simulink model "JointSpaceControl_BestInertia"  (R2013a)
settings: Solver=ode3  StartTime=0.0  StopTime=sim_end  FixedStep=0.004  MaxStep=0.008  RelTol=1e-3
PreLoadFcn:
  | Initialization
InitFcn:
  | Initialization
values from neighbouring files (symbols this model uses):
  a_max = [27 27 27 27 27 27]    [Initialization.m]
  dq_0 = qd_actual.signals.values(1,:)    [Initialization.m]
  K_0 = [K0_11, zeros(3,3); zeros(3,3),omega_P_small^2*eye(3,3)]    [Initialization.m]    (also in Plot_PD_Estimation.m)
  K_1 = [K1_11, zeros(3,3); zeros(3,3),2*omega_D_small*eye(3,3)]    [Initialization.m]    (also in Plot_PD_Estimation.m)
  q_0 = q_actual.signals.values(1,:)    [Initialization.m]
  q_max = 2*pi*ones(1,6)    [Initialization.m]
  q_min = -2*pi*ones(1,6)    [Initialization.m]
  torque_max = [150 150 150 28 28 28]    [Initialization.m]
  v_max = 3.4*ones(1,6)    [Initialization.m]
libraries: dsparch4 x30, simulink x2
(part 2 of 3)

== matlab function JointSpaceControl_BestInertia/base_tool_transformation_matrix1 ==
  data: d output; q input; R output
function [d, R]   = base_tool_transformation(q)
% BASE_TOOL_TRANSFORMATION - Transformationmatrix from Base to Tool.
%  Calculates the Base-Tool Transformation matrix based on the current
%  joint positions and returns the rotation matrix and the displacement
%  vector.

theta1 = q(1);
theta2 = q(2);
theta3 = q(3);
theta4 = q(4);
theta5 = q(5);
theta6 = q(6);

theta_1 = theta1;
theta_2 = theta2;
theta_3 = theta3;
theta_4 = theta4;
theta_5 = theta5;
theta_6 = theta6;

% With transformation to accelerometer
T = [[   cos(theta_6)*(sin(theta_1)*sin(theta_5) - cos(theta_5)*(cos(theta_4)*(cos(theta_1)*sin(theta_2)*sin(theta_3) - cos(theta_1)*cos(theta_2)*cos(theta_3)) + sin(theta_4)*(cos(theta_1)*cos(theta_2)*sin(theta_3) + cos(theta_1)*cos(theta_3)*sin(theta_2)))) - sin(theta_6)*(cos(theta_4)*(cos(theta_1)*cos(theta_2)*sin(theta_3) + cos(theta_1)*cos(theta_3)*sin(theta_2)) - sin(theta_4)*(cos(theta_1)*sin(theta_2)*sin(theta_3) - cos(theta_1)*cos(theta_2)*cos(theta_3))), - sin(theta_6)*(sin(theta_1)*sin(theta_5) - cos(theta_5)*(cos(theta_4)*(cos(theta_1)*sin(theta_2)*sin(theta_3) - cos(theta_1)*cos(theta_2)*cos(theta_3)) + sin(theta_4)*(cos(theta_1)*cos(theta_2)*sin(theta_3) + cos(theta_1)*cos(theta_3)*sin(theta_2)))) - cos(theta_6)*(cos(theta_4)*(cos(theta_1)*cos(theta_2)*sin(theta_3) + cos(theta_1)*cos(theta_3)*sin(theta_2)) - sin(theta_4)*(cos(theta_1)*sin(theta_2)*sin(theta_3) - cos(theta_1)*cos(theta_2)*cos(theta_3))), cos(theta_5)*sin(theta_1) + sin(theta_5)*(cos(theta_4)*(cos(theta_1)*sin(theta_2)*sin(theta_3) - cos(theta_1)*cos(theta_2)*cos(theta_3)) + sin(theta_4)*(cos(theta_1)*cos(theta_2)*sin(theta_3) + cos(theta_1)*cos(theta_3)*sin(theta_2))), (109*sin(theta_1))/1000 - (17*cos(theta_1)*cos(theta_2))/40 + (183*cos(theta_5)*sin(theta_1))/2000 + (347*cos(theta_6)*(sin(theta_1)*sin(theta_5) - cos(theta_5)*(cos(theta_4)*(cos(theta_1)*sin(theta_2)*sin(theta_3) - cos(theta_1)*cos(theta_2)*cos(theta_3)) + sin(theta_4)*(cos(theta_1)*cos(theta_2)*sin(theta_3) + cos(theta_1)*cos(theta_3)*sin(theta_2)))))/20000 + (93*cos(theta_4)*(cos(theta_1)*cos(theta_2)*sin(theta_3) + cos(theta_1)*cos(theta_3)*sin(theta_2)))/1000 - (121*sin(theta_6)*(sin(theta_1)*sin(theta_5) - cos(theta_5)*(cos(theta_4)*(cos(theta_1)*sin(theta_2)*sin(theta_3) - cos(theta_1)*cos(theta_2)*cos(theta_3)) + sin(theta_4)*(cos(theta_1)*cos(theta_2)*sin(theta_3) + cos(theta_1)*cos(theta_3)*sin(theta_2)))))/20000 - (93*sin(theta_4)*(cos(theta_1)*sin(theta_2)*sin(theta_3) - cos(theta_1)*cos(theta_2)*cos(theta_3)))/1000 - (121*cos(theta_6)*(cos(theta_4)*(cos(theta_1)*cos(theta_2)*sin(theta_3) + cos(theta_1)*cos(theta_3)*sin(theta_2)) - sin(theta_4)*(cos(theta_1)*sin(theta_2)*sin(theta_3) - cos(theta_1)*cos(theta_2)*cos(theta_3))))/20000 + (183*sin(theta_5)*(cos(theta_4)*(cos(theta_1)*sin(theta_2)*sin(theta_3) - cos(theta_1)*cos(theta_2)*cos(theta_3)) + sin(theta_4)*(cos(theta_1)*cos(theta_2)*sin(theta_3) + cos(theta_1)*cos(theta_3)*sin(theta_2))))/2000 - (347*sin(theta_6)*(cos(theta_4)*(cos(theta_1)*cos(theta_2)*sin(theta_3) + cos(theta_1)*cos(theta_3)*sin(theta_2)) - sin(theta_4)*(cos(theta_1)*sin(theta_2)*sin(theta_3) - cos(theta_1)*cos(theta_2)*cos(theta_3))))/20000 + (39243*cos(theta_1)*sin(theta_2)*sin(theta_3))/100000 - (39243*cos(theta_1)*cos(theta_2)*cos(theta_3))/100000]; 
    [ - cos(theta_6)*(cos(theta_1)*sin(theta_5) + cos(theta_5)*(cos(theta_4)*(sin(theta_1)*sin(theta_2)*sin(theta_3) - cos(theta_2)*cos(theta_3)*sin(theta_1)) + sin(theta_4)*(cos(theta_2)*sin(theta_1)*sin(theta_3) + cos(theta_3)*sin(theta_1)*sin(theta_2)))) - sin(theta_6)*(cos(theta_4)*(cos(theta_2)*sin(theta_1)*sin(theta_3) + cos(theta_3)*sin(theta_1)*sin(theta_2)) - sin(theta_4)*(sin(theta_1)*sin(theta_2)*sin(theta_3) - cos(theta_2)*cos(theta_3)*sin(theta_1))),   sin(theta_6)*(cos(theta_1)*sin(theta_5) + cos(theta_5)*(cos(theta_4)*(sin(theta_1)*sin(theta_2)*sin(theta_3) - cos(theta_2)*cos(theta_3)*sin(theta_1)) + sin(theta_4)*(cos(theta_2)*sin(theta_1)*sin(theta_3) + cos(theta_3)*sin(theta_1)*sin(theta_2)))) - cos(theta_6)*(cos(theta_4)*(cos(theta_2)*sin(theta_1)*sin(theta_3) + cos(theta_3)*sin(theta_1)*sin(theta_2)) - sin(theta_4)*(sin(theta_1)*sin(theta_2)*sin(theta_3) - cos(theta_2)*cos(theta_3)*sin(theta_1))), sin(theta_5)*(cos(theta_4)*(sin(theta_1)*sin(theta_2)*sin(theta_3) - cos(theta_2)*cos(theta_3)*sin(theta_1)) + sin(theta_4)*(cos(theta_2)*sin(theta_1)*sin(theta_3) + cos(theta_3)*sin(theta_1)*sin(theta_2))) - cos(theta_1)*cos(theta_5), (93*cos(theta_4)*(cos(theta_2)*sin(theta_1)*sin(theta_3) + cos(theta_3)*sin(theta_1)*sin(theta_2)))/1000 - (183*cos(theta_1)*cos(theta_5))/2000 - (17*cos(theta_2)*sin(theta_1))/40 - (109*cos(theta_1))/1000 - (347*cos(theta_6)*(cos(theta_1)*sin(theta_5) + cos(theta_5)*(cos(theta_4)*(sin(theta_1)*sin(theta_2)*sin(theta_3) - cos(theta_2)*cos(theta_3)*sin(theta_1)) + sin(theta_4)*(cos(theta_2)*sin(theta_1)*sin(theta_3) + cos(theta_3)*sin(theta_1)*sin(theta_2)))))/20000 - (93*sin(theta_4)*(sin(theta_1)*sin(theta_2)*sin(theta_3) - cos(theta_2)*cos(theta_3)*sin(theta_1)))/1000 + (121*sin(theta_6)*(cos(theta_1)*sin(theta_5) + cos(theta_5)*(cos(theta_4)*(sin(theta_1)*sin(theta_2)*sin(theta_3) - cos(theta_2)*cos(theta_3)*sin(theta_1)) + sin(theta_4)*(cos(theta_2)*sin(theta_1)*sin(theta_3) + cos(theta_3)*sin(theta_1)*sin(theta_2)))))/20000 - (121*cos(theta_6)*(cos(theta_4)*(cos(theta_2)*sin(theta_1)*sin(theta_3) + cos(theta_3)*sin(theta_1)*sin(theta_2)) - sin(theta_4)*(sin(theta_1)*sin(theta_2)*sin(theta_3) - cos(theta_2)*cos(theta_3)*sin(theta_1))))/20000 + (183*sin(theta_5)*(cos(theta_4)*(sin(theta_1)*sin(theta_2)*sin(theta_3) - cos(theta_2)*cos(theta_3)*sin(theta_1)) + sin(theta_4)*(cos(theta_2)*sin(theta_1)*sin(theta_3) + cos(theta_3)*sin(theta_1)*sin(theta_2))))/2000 - (347*sin(theta_6)*(cos(theta_4)*(cos(theta_2)*sin(theta_1)*sin(theta_3) + cos(theta_3)*sin(theta_1)*sin(theta_2)) - sin(theta_4)*(sin(theta_1)*sin(theta_2)*sin(theta_3) - cos(theta_2)*cos(theta_3)*sin(theta_1))))/20000 + (39243*sin(theta_1)*sin(theta_2)*sin(theta_3))/100000 - (39243*cos(theta_2)*cos(theta_3)*sin(theta_1))/100000]; 
    [                                                                                                                                         sin(theta_6)*(cos(theta_4)*(cos(theta_2)*cos(theta_3) - sin(theta_2)*sin(theta_3)) - sin(theta_4)*(cos(theta_2)*sin(theta_3) + cos(theta_3)*sin(theta_2))) + cos(theta_5)*cos(theta_6)*(cos(theta_4)*(cos(theta_2)*sin(theta_3) + cos(theta_3)*sin(theta_2)) + sin(theta_4)*(cos(theta_2)*cos(theta_3) - sin(theta_2)*sin(theta_3))),                                                                                                                                         cos(theta_6)*(cos(theta_4)*(cos(theta_2)*cos(theta_3) - sin(theta_2)*sin(theta_3)) - sin(theta_4)*(cos(theta_2)*sin(theta_3) + cos(theta_3)*sin(theta_2))) - cos(theta_5)*sin(theta_6)*(cos(theta_4)*(cos(theta_2)*sin(theta_3) + cos(theta_3)*sin(theta_2)) + sin(theta_4)*(cos(theta_2)*cos(theta_3) - sin(theta_2)*sin(theta_3))),                                                                                -sin(theta_5)*(cos(theta_4)*(cos(theta_2)*sin(theta_3) + cos(theta_3)*sin(theta_2)) + sin(theta_4)*(cos(theta_2)*cos(theta_3) - sin(theta_2)*sin(theta_3))),                                                                                                                                                                                                                                                                                                                                                                                                                                                                                  (121*cos(theta_6)*(cos(theta_4)*(cos(theta_2)*cos(theta_3) - sin(theta_2)*sin(theta_3)) - sin(theta_4)*(cos(theta_2)*sin(theta_3) + cos(theta_3)*sin(theta_2))))/20000 - (39243*cos(theta_2)*sin(theta_3))/100000 - (39243*cos(theta_3)*sin(theta_2))/100000 - (17*sin(theta_2))/40 - (183*sin(theta_5)*(cos(theta_4)*(cos(theta_2)*sin(theta_3) + cos(theta_3)*sin(theta_2)) + sin(theta_4)*(cos(theta_2)*cos(theta_3) - sin(theta_2)*sin(theta_3))))/2000 + (347*sin(theta_6)*(cos(theta_4)*(cos(theta_2)*cos(theta_3) - sin(theta_2)*sin(theta_3)) - sin(theta_4)*(cos(theta_2)*sin(theta_3) + cos(theta_3)*sin(theta_2))))/20000 - (93*cos(theta_4)*(cos(theta_2)*cos(theta_3) - sin(theta_2)*sin(theta_3)))/1000 + (93*sin(theta_4)*(cos(theta_2)*sin(theta_3) + cos(theta_3)*sin(theta_2)))/1000 + (347*cos(theta_5)*cos(theta_6)*(cos(theta_4)*(cos(theta_2)*sin(theta_3) + cos(theta_3)*sin(theta_2)) + sin(theta_4)*(cos(theta_2)*cos(theta_3) - sin(theta_2)*sin(theta_3))))/20000 - (121*cos(theta_5)*sin(theta_6)*(cos(theta_4)*(cos(theta_2)*sin(theta_3) + cos(theta_3)*sin(theta_2)) + sin(theta_4)*(cos(theta_2)*cos(theta_3) - sin(theta_2)*sin(theta_3))))/20000 + 223/2500]; 
    [                                                                                                                                                                                                                                                                                                                                                                                                                                                                            0,                                                                                                                                                                                                                                                                                                                                                                                                                                                                            0,                                                                                                                                                                                                                                          0,                                                                                                                                                                                                                                                                                                                                                                                                                                                                                                                                                                                                                                                                                                                                                                                                                                                                                                                                                                                                                                                                                                                                                                                                                                                                                                                                                                                                                                                                                                                                                                                                                                                                              1]];


% T =  [[cos(theta_6)*(sin(theta_1)*sin(theta_5) - cos(theta_5)*(cos(theta_4)*(cos(theta_1)*sin(theta_2)*sin(theta_3) - cos(theta_1)*cos(theta_2)*cos(theta_3)) + sin(theta_4)*(cos(theta_1)*cos(theta_2)*sin(theta_3) + cos(theta_1)*cos(theta_3)*sin(theta_2)))) - sin(theta_6)*(cos(theta_4)*(cos(theta_1)*cos(theta_2)*sin(theta_3) + cos(theta_1)*cos(theta_3)*sin(theta_2)) - sin(theta_4)*(cos(theta_1)*sin(theta_2)*sin(theta_3) - cos(theta_1)*cos(theta_2)*cos(theta_3))), - sin(theta_6)*(sin(theta_1)*sin(theta_5) - cos(theta_5)*(cos(theta_4)*(cos(theta_1)*sin(theta_2)*sin(theta_3) - cos(theta_1)*cos(theta_2)*cos(theta_3)) + sin(theta_4)*(cos(theta_1)*cos(theta_2)*sin(theta_3) + cos(theta_1)*cos(theta_3)*sin(theta_2)))) - cos(theta_6)*(cos(theta_4)*(cos(theta_1)*cos(theta_2)*sin(theta_3) + cos(theta_1)*cos(theta_3)*sin(theta_2)) - sin(theta_4)*(cos(theta_1)*sin(theta_2)*sin(theta_3) - cos(theta_1)*cos(theta_2)*cos(theta_3))), cos(theta_5)*sin(theta_1) + sin(theta_5)*(cos(theta_4)*(cos(theta_1)*sin(theta_2)*sin(theta_3) - cos(theta_1)*cos(theta_2)*cos(theta_3)) + sin(theta_4)*(cos(theta_1)*cos(theta_2)*sin(theta_3) + cos(theta_1)*cos(theta_3)*sin(theta_2))), (109*sin(theta_1))/1000 - (17*cos(theta_1)*cos(theta_2))/40 + (41*cos(theta_5)*sin(theta_1))/500 + (93*cos(theta_4)*(cos(theta_1)*cos(theta_2)*sin(theta_3) + cos(theta_1)*cos(theta_3)*sin(theta_2)))/1000 - (93*sin(theta_4)*(cos(theta_1)*sin(theta_2)*sin(theta_3) - cos(theta_1)*cos(theta_2)*cos(theta_3)))/1000 + (41*sin(theta_5)*(cos(theta_4)*(cos(theta_1)*sin(theta_2)*sin(theta_3) - cos(theta_1)*cos(theta_2)*cos(theta_3)) + sin(theta_4)*(cos(theta_1)*cos(theta_2)*sin(theta_3) + cos(theta_1)*cos(theta_3)*sin(theta_2))))/500 + (39243*cos(theta_1)*sin(theta_2)*sin(theta_3))/100000 - (39243*cos(theta_1)*cos(theta_2)*cos(theta_3))/100000];
%      [ - cos(theta_6)*(cos(theta_1)*sin(theta_5) + cos(theta_5)*(cos(theta_4)*(sin(theta_1)*sin(theta_2)*sin(theta_3) - cos(theta_2)*cos(theta_3)*sin(theta_1)) + sin(theta_4)*(cos(theta_2)*sin(theta_1)*sin(theta_3) + cos(theta_3)*sin(theta_1)*sin(theta_2)))) - sin(theta_6)*(cos(theta_4)*(cos(theta_2)*sin(theta_1)*sin(theta_3) + cos(theta_3)*sin(theta_1)*sin(theta_2)) - sin(theta_4)*(sin(theta_1)*sin(theta_2)*sin(theta_3) - cos(theta_2)*cos(theta_3)*sin(theta_1))),   sin(theta_6)*(cos(theta_1)*sin(theta_5) + cos(theta_5)*(cos(theta_4)*(sin(theta_1)*sin(theta_2)*sin(theta_3) - cos(theta_2)*cos(theta_3)*sin(theta_1)) + sin(theta_4)*(cos(theta_2)*sin(theta_1)*sin(theta_3) + cos(theta_3)*sin(theta_1)*sin(theta_2)))) - cos(theta_6)*(cos(theta_4)*(cos(theta_2)*sin(theta_1)*sin(theta_3) + cos(theta_3)*sin(theta_1)*sin(theta_2)) - sin(theta_4)*(sin(theta_1)*sin(theta_2)*sin(theta_3) - cos(theta_2)*cos(theta_3)*sin(theta_1))), sin(theta_5)*(cos(theta_4)*(sin(theta_1)*sin(theta_2)*sin(theta_3) - cos(theta_2)*cos(theta_3)*sin(theta_1)) + sin(theta_4)*(cos(theta_2)*sin(theta_1)*sin(theta_3) + cos(theta_3)*sin(theta_1)*sin(theta_2))) - cos(theta_1)*cos(theta_5), (93*cos(theta_4)*(cos(theta_2)*sin(theta_1)*sin(theta_3) + cos(theta_3)*sin(theta_1)*sin(theta_2)))/1000 - (41*cos(theta_1)*cos(theta_5))/500 - (17*cos(theta_2)*sin(theta_1))/40 - (109*cos(theta_1))/1000 - (93*sin(theta_4)*(sin(theta_1)*sin(theta_2)*sin(theta_3) - cos(theta_2)*cos(theta_3)*sin(theta_1)))/1000 + (41*sin(theta_5)*(cos(theta_4)*(sin(theta_1)*sin(theta_2)*sin(theta_3) - cos(theta_2)*cos(theta_3)*sin(theta_1)) + sin(theta_4)*(cos(theta_2)*sin(theta_1)*sin(theta_3) + cos(theta_3)*sin(theta_1)*sin(theta_2))))/500 + (39243*sin(theta_1)*sin(theta_2)*sin(theta_3))/100000 - (39243*cos(theta_2)*cos(theta_3)*sin(theta_1))/100000];
%      [                                                                                                                                         sin(theta_6)*(cos(theta_4)*(cos(theta_2)*cos(theta_3) - sin(theta_2)*sin(theta_3)) - sin(theta_4)*(cos(theta_2)*sin(theta_3) + cos(theta_3)*sin(theta_2))) + cos(theta_5)*cos(theta_6)*(cos(theta_4)*(cos(theta_2)*sin(theta_3) + cos(theta_3)*sin(theta_2)) + sin(theta_4)*(cos(theta_2)*cos(theta_3) - sin(theta_2)*sin(theta_3))),                                                                                                                                         cos(theta_6)*(cos(theta_4)*(cos(theta_2)*cos(theta_3) - sin(theta_2)*sin(theta_3)) - sin(theta_4)*(cos(theta_2)*sin(theta_3) + cos(theta_3)*sin(theta_2))) - cos(theta_5)*sin(theta_6)*(cos(theta_4)*(cos(theta_2)*sin(theta_3) + cos(theta_3)*sin(theta_2)) + sin(theta_4)*(cos(theta_2)*cos(theta_3) - sin(theta_2)*sin(theta_3))),                                                                                -sin(theta_5)*(cos(theta_4)*(cos(theta_2)*sin(theta_3) + cos(theta_3)*sin(theta_2)) + sin(theta_4)*(cos(theta_2)*cos(theta_3) - sin(theta_2)*sin(theta_3))),                                                                                                                                                                                                    (93*sin(theta_4)*(cos(theta_2)*sin(theta_3) + cos(theta_3)*sin(theta_2)))/1000 - (39243*cos(theta_2)*sin(theta_3))/100000 - (39243*cos(theta_3)*sin(theta_2))/100000 - (41*sin(theta_5)*(cos(theta_4)*(cos(theta_2)*sin(theta_3) + cos(theta_3)*sin(theta_2)) + sin(theta_4)*(cos(theta_2)*cos(theta_3) - sin(theta_2)*sin(theta_3))))/500 - (93*cos(theta_4)*(cos(theta_2)*cos(theta_3) - sin(theta_2)*sin(theta_3)))/1000 - (17*sin(theta_2))/40 + 223/2500];
%      [                                                                                                                                                                                                                                                                                                                                                                                                                                                                            0,                                                                                                                                                                                                                                                                                                                                                                                                                                                                            0,                                                                                                                                                                                                                                          0,                                                                                                                                                                                                                                                                                                                                                                                                                                                                                                                                                                                                                                                                1]];


% 
% T = [(((cos(theta1) * cos(theta2) * cos(theta3) - cos(theta1) * sin(theta2) ...
%     * sin(theta3)) * cos(theta4) + (-cos(theta1) * cos(theta2) * sin(theta3) ...
%     - cos(theta1) * sin(theta2) * cos(theta3)) * sin(theta4)) * cos(theta5) ...
%     + sin(theta1) * sin(theta5)) * cos(theta6) + (-(cos(theta1) * cos(theta2) ...
%     * cos(theta3) - cos(theta1) * sin(theta2) * sin(theta3)) * sin(theta4) + ...
%     (-cos(theta1) * cos(theta2) * sin(theta3) - cos(theta1) * sin(theta2) * ...
%     cos(theta3)) * cos(theta4)) * sin(theta6) -(((cos(theta1) * cos(theta2) * ...
%     cos(theta3) - cos(theta1) * sin(theta2) * sin(theta3)) * cos(theta4) + ...
%     (-cos(theta1) * cos(theta2) * sin(theta3) - cos(theta1) * sin(theta2) * ...
%     cos(theta3)) * sin(theta4)) * cos(theta5) + sin(theta1) * sin(theta5)) * ...
%     sin(theta6) + (-(cos(theta1) * cos(theta2) * cos(theta3) - cos(theta1) * ...
%     sin(theta2) * sin(theta3)) * sin(theta4) + (-cos(theta1) * cos(theta2) * ...
%     sin(theta3) - cos(theta1) * sin(theta2) * cos(theta3)) * cos(theta4)) * ...
%     cos(theta6) -((cos(theta1) * cos(theta2) * cos(theta3) - cos(theta1) * ...
%     sin(theta2) * sin(theta3)) * cos(theta4) + (-cos(theta1) * cos(theta2) * ...
%     sin(theta3) - cos(theta1) * sin(theta2) * cos(theta3)) * sin(theta4)) * ...
%     sin(theta5) + sin(theta1) * cos(theta5) -0.082 * ((cos(theta1) * ...
%     cos(theta2) * cos(theta3) - cos(theta1) * sin(theta2) * sin(theta3)) * ...
%     cos(theta4) + (-cos(theta1) * cos(theta2) * sin(theta3) - cos(theta1) * ...
%     sin(theta2) * cos(theta3)) * sin(theta4)) * sin(theta5) + 0.082 * ...
%     sin(theta1) * cos(theta5) + 0.093 * (cos(theta1) * cos(theta2) * ...
%     cos(theta3) - cos(theta1) * sin(theta2) * sin(theta3)) * sin(theta4) - ...
%     0.093 * (-cos(theta1) * cos(theta2) * sin(theta3) - cos(theta1) * ...
%     sin(theta2) * cos(theta3)) * cos(theta4) + 0.109 * sin(theta1) - ...
%     0.39243 * cos(theta1) * cos(theta2) * cos(theta3) + 0.39243 * ...
%     cos(theta1) * sin(theta2) * sin(theta3) - 0.425 * cos(theta1) * cos(theta2); ...
%     (((sin(theta1) * cos(theta2) * cos(theta3) - sin(theta1) * sin(theta2) * ...
%     sin(theta3)) * cos(theta4) + (-sin(theta1) * cos(theta2) * sin(theta3) - ...
%     sin(theta1) * sin(theta2) * cos(theta3)) * sin(theta4)) * cos(theta5) - ...
%     cos(theta1) * sin(theta5)) * cos(theta6) + (-(sin(theta1) * cos(theta2) * ...
%     cos(theta3) - sin(theta1) * sin(theta2) * sin(theta3)) * sin(theta4) + ...
%     (-sin(theta1) * cos(theta2) * sin(theta3) - sin(theta1) * sin(theta2) * ...
%     cos(theta3)) * cos(theta4)) * sin(theta6) -(((sin(theta1) * cos(theta2) *...
%     cos(theta3) - sin(theta1) * sin(theta2) * sin(theta3)) * cos(theta4) + ...
%     (-sin(theta1) * cos(theta2) * sin(theta3) - sin(theta1) * sin(theta2) * ...
%     cos(theta3)) * sin(theta4)) * cos(theta5) - cos(theta1) * sin(theta5)) * ...
%     sin(theta6) + (-(sin(theta1) * cos(theta2) * cos(theta3) - sin(theta1) * ...
%     sin(theta2) * sin(theta3)) * sin(theta4) + (-sin(theta1) * cos(theta2) * ...
%     sin(theta3) - sin(theta1) * sin(theta2) * cos(theta3)) * cos(theta4)) * ...
%     cos(theta6) -((sin(theta1) * cos(theta2) * cos(theta3) - sin(theta1) * ...
%     sin(theta2) * sin(theta3)) * cos(theta4) + (-sin(theta1) * cos(theta2) * ...
%     sin(theta3) - sin(theta1) * sin(theta2) * cos(theta3)) * sin(theta4)) *...
%      sin(theta5) - cos(theta1) * cos(theta5) -0.082 * ((sin(theta1) * ...
%     cos(theta2) * cos(theta3) - sin(theta1) * sin(theta2) * sin(theta3)) * ...
%     cos(theta4) + (-sin(theta1) * cos(theta2) * sin(theta3) - sin(theta1) * ...
%     sin(theta2) * cos(theta3)) * sin(theta4)) * sin(theta5) - 0.082 * ...
%     cos(theta1) * cos(theta5) + 0.093 * (sin(theta1) * cos(theta2) * ...
%     cos(theta3) - sin(theta1) * sin(theta2) * sin(theta3)) * sin(theta4) - ...
%     0.093 * (-sin(theta1) * cos(theta2) * sin(theta3) - sin(theta1) * ...
%     sin(theta2) * cos(theta3)) * cos(theta4) - 0.109 * cos(theta1) - ...
%     0.39243 * sin(theta1) * cos(theta2) * cos(theta3) + 0.39243 * ...
%     sin(theta1) * sin(theta2) * sin(theta3) - 0.425 * sin(theta1) * ...
%     cos(theta2); ((sin(theta2) * cos(theta3) + cos(theta2) * sin(theta3)) ...
%     * cos(theta4) + (-sin(theta2) * sin(theta3) + cos(theta2) * cos(theta3)) ...
%     * sin(theta4)) * cos(theta5) * cos(theta6) + (-(sin(theta2) * cos(theta3) ...
%     + cos(theta2) * sin(theta3)) * sin(theta4) + (-sin(theta2) * sin(theta3) ...
%     + cos(theta2) * cos(theta3)) * cos(theta4)) * sin(theta6) -((sin(theta2) ...
%     * cos(theta3) + cos(theta2) * sin(theta3)) * cos(theta4) + (-sin(theta2) ...
%     * sin(theta3) + cos(theta2) * cos(theta3)) * sin(theta4)) * cos(theta5) ...
%     * sin(theta6) + (-(sin(theta2) * cos(theta3) + cos(theta2) * sin(theta3)) ...
%     * sin(theta4) + (-sin(theta2) * sin(theta3) + cos(theta2) * cos(theta3)) ...
%     * cos(theta4)) * cos(theta6) -((sin(theta2) * cos(theta3) + cos(theta2) ...
%     * sin(theta3)) * cos(theta4) + (-sin(theta2) * sin(theta3) + cos(theta2) ...
%     * cos(theta3)) * sin(theta4)) * sin(theta5) 0.0892 - 0.082 * ...
%     ((sin(theta2) * cos(theta3) + cos(theta2) * sin(theta3)) * cos(theta4) ...
%     + (-sin(theta2) * sin(theta3) + cos(theta2) * cos(theta3)) * sin(theta4)) ...
%     * sin(theta5) + 0.093 * (sin(theta2) * cos(theta3) + cos(theta2) * ...
%     sin(theta3)) * sin(theta4) - 0.093 * (-sin(theta2) * sin(theta3) + ...
%     cos(theta2) * cos(theta3)) * cos(theta4) - 0.39243 * sin(theta2) * ...
%     cos(theta3) - 0.39243 * cos(theta2) * sin(theta3) - 0.425 * sin(theta2); ...
%     0 0 0 1;];

R = T(1:3,1:3);
d = T(1:3,4);

end

== matlab function JointSpaceControl_BestInertia/Forward & Velocity Kinematics Joint -> Tool Geometric Jacobian/R -> Euler ==
  data: theta output; phi output; R input; psi output
function [theta, phi, psi]  = R_to_euler_angle(R)
%R_TO_EULER_ANGLE Transform rotation matrix to euler-angle format, where
%the rotation happens around ZYZ, with R_ZYZ = R_Z,phi*R_Y,theta*R_Z,psi
r_11 = R(1,1);
r_12 = R(1,2);
r_13 = R(1,3);
r_21 = R(2,1);
r_22 = R(2,2);
r_23 = R(2,3);
r_31 = R(3,1);
r_32 = R(3,2);
r_33 = R(3,3);

if (r_13 ~= 0) || (r_23 ~= 0)
    theta = atan2(sqrt(r_13^2+r_23^2),r_33);
    phi = atan2(r_23, r_13);
    psi = atan2(r_32, -r_31);
elseif (r_13 == 0) && (r_23 == 0)
    if (r_33 == 1)
        theta = 0;
        phi = 0;
        psi = atan2(r_11, r_21) - phi;
    elseif (r_33 == -1)
        theta = pi;
        phi = 0;
        psi = -(atan2(-r_11, -r_12) - phi);
    else
        error('r_33 must be +1 or -1')
    end
else
    error('Make sure that the values are almost equal zero')
end
end

== matlab function JointSpaceControl_BestInertia/Forward & Velocity Kinematics Joint -> Tool Geometric Jacobian/transformation_matrix_to_axis_angle ==
  data: k output; R input; theta output
function [k, theta]  = R_to_axis_angle(R)
%BaseToolTransformationMatrix - Transformationmatrix from Base to Tool
%  Calculates the Base-Tool Transformation matrix based on the current
%  joint positions.
 theta = acos((R(1,1)+R(2,2)+R(3,3)-1)/2);
 k = 1/(2*sin(theta))*[R(3,2)-R(2,3); R(1,3)-R(3,1); R(2,1)-R(1,2)];
end

== matlab function JointSpaceControl_BestInertia/RxRyRz to axis angle ==
  data: RxRyRz input; k output; theta output
function [k, theta]  = RxRyRz_to_k_theta(RxRyRz)
% RXRYRZ_TO_K_THETA Transform the RxRyRz representation to the axis/angle
% representation
 theta = norm(RxRyRz);
 k = RxRyRz/theta;
end

== matlab function JointSpaceControl_BestInertia/axis angle to transformation matrix ==
  data: k input; theta input; R output
function R   = axis_angle_to_R(k, theta)
% AXIS_ANGLE_TO_R Transform the axis/angle representation to a rotation
% matrix representation.
kx = k(1);
ky = k(2);
kz = k(3);

v = 1-cos(theta);
s = sin(theta);
c = cos (theta);

r11 = kx^2*v + c;
r12 = kx*ky*v - kz*s;
r13 = kx*kz*v+ky*s;
r21 = kx*ky*v+kz*s;
r22 = ky^2*v + c;
r23 = ky*kz*v-kx*s;
r31 = kx*kz*v-ky*s;
r32 = ky*kz*v + kx*s;
r33 = kz^2*v+c;

R = [r11, r12, r13; r21, r22, r23; r31, r32, r33];

end

== matlab function JointSpaceControl_BestInertia/Forward & Velocity Kinematics Joint -> Tool Geometric Jacobian/tcp_speed (by using Jacobian) ==
  data: tcp_speed output; q input; dq input
function tcp_speed     = tcp_speed(q, dq)
% JACOBIAN - Jacobian from Base to Tool.
%  Calculates the Base-Tool Transformation matrix based on the current
%  joint positions and returns the rotation matrix and the displacement
%  vector.

theta_1 = q(1);
theta_2 = q(2);
theta_3 = q(3);
theta_4 = q(4);
theta_5 = q(5);
theta_6 = q(6);

J = [(109*cos(theta_1))/1000 + (41*cos(theta_1)*cos(theta_5))/500 + ...
        (17*cos(theta_2)*sin(theta_1))/40 - ...
        (93*cos(theta_4)*(cos(theta_2)*sin(theta_1)*sin(theta_3) + ...
        cos(theta_3)*sin(theta_1)*sin(theta_2)))/1000 + ...
        (93*sin(theta_4)*(sin(theta_1)*sin(theta_2)*sin(theta_3) - ...
        cos(theta_2)*cos(theta_3)*sin(theta_1)))/1000 - ...
        (41*sin(theta_5)*(cos(theta_4)*(sin(theta_1)*sin(theta_2)*sin(theta_3) - ...
        cos(theta_2)*cos(theta_3)*sin(theta_1)) + ...
        sin(theta_4)*(cos(theta_2)*sin(theta_1)*sin(theta_3) + ...
        cos(theta_3)*sin(theta_1)*sin(theta_2))))/500 - ...
        (39243*sin(theta_1)*sin(theta_2)*sin(theta_3))/100000 + ...
        (39243*cos(theta_2)*cos(theta_3)*sin(theta_1))/100000, ...
        ...
        (17*cos(theta_1)*sin(theta_2))/40 - ...
        (93*cos(theta_4)*(cos(theta_1)*sin(theta_2)*sin(theta_3) - ...
        cos(theta_1)*cos(theta_2)*cos(theta_3)))/1000 - ...
        (93*sin(theta_4)*(cos(theta_1)*cos(theta_2)*sin(theta_3) + ...
        cos(theta_1)*cos(theta_3)*sin(theta_2)))/1000 + ...
        (41*sin(theta_5)*(cos(theta_4)*(cos(theta_1)*cos(theta_2)*sin(theta_3) + ...
        cos(theta_1)*cos(theta_3)*sin(theta_2)) - ...
        sin(theta_4)*(cos(theta_1)*sin(theta_2)*sin(theta_3) - ...
        cos(theta_1)*cos(theta_2)*cos(theta_3))))/500 + ...
        (39243*cos(theta_1)*cos(theta_2)*sin(theta_3))/100000 + ...
        (39243*cos(theta_1)*cos(theta_3)*sin(theta_2))/100000, ...
        ...
        (41*sin(theta_5)*(cos(theta_4)*(cos(theta_1)*cos(theta_2)*sin(theta_3) + ...
        cos(theta_1)*cos(theta_3)*sin(theta_2)) - ...
        sin(theta_4)*(cos(theta_1)*sin(theta_2)*sin(theta_3) - ...
        cos(theta_1)*cos(theta_2)*cos(theta_3))))/500 - ...
        (93*sin(theta_4)*(cos(theta_1)*cos(theta_2)*sin(theta_3) + ...
        cos(theta_1)*cos(theta_3)*sin(theta_2)))/1000 - ...
        (93*cos(theta_4)*(cos(theta_1)*sin(theta_2)*sin(theta_3) - ...
        cos(theta_1)*cos(theta_2)*cos(theta_3)))/1000 + ...
        (39243*cos(theta_1)*cos(theta_2)*sin(theta_3))/100000 + ...
        (39243*cos(theta_1)*cos(theta_3)*sin(theta_2))/100000, ...
        ...
        (41*sin(theta_5)*(cos(theta_4)*(cos(theta_1)*cos(theta_2)*sin(theta_3) + ...
        cos(theta_1)*cos(theta_3)*sin(theta_2)) - ...
        sin(theta_4)*(cos(theta_1)*sin(theta_2)*sin(theta_3) - ...
        cos(theta_1)*cos(theta_2)*cos(theta_3))))/500 - ...
        (93*sin(theta_4)*(cos(theta_1)*cos(theta_2)*sin(theta_3) + ...
        cos(theta_1)*cos(theta_3)*sin(theta_2)))/1000 - ...
        (93*cos(theta_4)*(cos(theta_1)*sin(theta_2)*sin(theta_3) - ...
        cos(theta_1)*cos(theta_2)*cos(theta_3)))/1000, ...
        ...
        (41*cos(theta_5)*(cos(theta_4)*(cos(theta_1)*sin(theta_2)*sin(theta_3) - ...
        cos(theta_1)*cos(theta_2)*cos(theta_3)) + ...
        sin(theta_4)*(cos(theta_1)*cos(theta_2)*sin(theta_3) + ...
        cos(theta_1)*cos(theta_3)*sin(theta_2))))/500 - ...
        (41*sin(theta_1)*sin(theta_5))/500,... 
        ...
        0; ...
   (109*sin(theta_1))/1000 - (17*cos(theta_1)*cos(theta_2))/40 + ...
        (41*cos(theta_5)*sin(theta_1))/500 + ...
        (93*cos(theta_4)*(cos(theta_1)*cos(theta_2)*sin(theta_3) + ...
        cos(theta_1)*cos(theta_3)*sin(theta_2)))/1000 - ...
        (93*sin(theta_4)*(cos(theta_1)*sin(theta_2)*sin(theta_3) - ... 
        cos(theta_1)*cos(theta_2)*cos(theta_3)))/1000 + ...
        (41*sin(theta_5)*(cos(theta_4)*(cos(theta_1)*sin(theta_2)*sin(theta_3) - ...
        cos(theta_1)*cos(theta_2)*cos(theta_3)) + ...
        sin(theta_4)*(cos(theta_1)*cos(theta_2)*sin(theta_3) + ...
        cos(theta_1)*cos(theta_3)*sin(theta_2))))/500 + ...
        (39243*cos(theta_1)*sin(theta_2)*sin(theta_3))/100000 - ...
        (39243*cos(theta_1)*cos(theta_2)*cos(theta_3))/100000, ...
        ...
        (17*sin(theta_1)*sin(theta_2))/40 - ...
        (93*cos(theta_4)*(sin(theta_1)*sin(theta_2)*sin(theta_3) - ...
        cos(theta_2)*cos(theta_3)*sin(theta_1)))/1000 - ...
        (93*sin(theta_4)*(cos(theta_2)*sin(theta_1)*sin(theta_3) + ...
        cos(theta_3)*sin(theta_1)*sin(theta_2)))/1000 + ...
        (41*sin(theta_5)*(cos(theta_4)*(cos(theta_2)*sin(theta_1)*sin(theta_3) + ...
        cos(theta_3)*sin(theta_1)*sin(theta_2)) - ...
        sin(theta_4)*(sin(theta_1)*sin(theta_2)*sin(theta_3) - ...
        cos(theta_2)*cos(theta_3)*sin(theta_1))))/500 + ...
        (39243*cos(theta_2)*sin(theta_1)*sin(theta_3))/100000 + ...
        (39243*cos(theta_3)*sin(theta_1)*sin(theta_2))/100000, ...
        ...
        (41*sin(theta_5)*(cos(theta_4)*(cos(theta_2)*sin(theta_1)*sin(theta_3) + ...
        cos(theta_3)*sin(theta_1)*sin(theta_2)) - ...
        sin(theta_4)*(sin(theta_1)*sin(theta_2)*sin(theta_3) - ...
        cos(theta_2)*cos(theta_3)*sin(theta_1))))/500 - ...
        (93*sin(theta_4)*(cos(theta_2)*sin(theta_1)*sin(theta_3) + ...
        cos(theta_3)*sin(theta_1)*sin(theta_2)))/1000 - ...
        (93*cos(theta_4)*(sin(theta_1)*sin(theta_2)*sin(theta_3) - ...
        cos(theta_2)*cos(theta_3)*sin(theta_1)))/1000 + ...
        (39243*cos(theta_2)*sin(theta_1)*sin(theta_3))/100000 + ...
        (39243*cos(theta_3)*sin(theta_1)*sin(theta_2))/100000, ...
        ...
        (41*sin(theta_5)*(cos(theta_4)*(cos(theta_2)*sin(theta_1)*sin(theta_3) + ...
        cos(theta_3)*sin(theta_1)*sin(theta_2)) - ...
        sin(theta_4)*(sin(theta_1)*sin(theta_2)*sin(theta_3) - ...
        cos(theta_2)*cos(theta_3)*sin(theta_1))))/500 - ...
        (93*sin(theta_4)*(cos(theta_2)*sin(theta_1)*sin(theta_3) + ...
        cos(theta_3)*sin(theta_1)*sin(theta_2)))/1000 - ...
        (93*cos(theta_4)*(sin(theta_1)*sin(theta_2)*sin(theta_3) - ...
        cos(theta_2)*cos(theta_3)*sin(theta_1)))/1000, ...
        ...
        (41*cos(theta_1)*sin(theta_5))/500 + ...
        (41*cos(theta_5)*(cos(theta_4)*(sin(theta_1)*sin(theta_2)*sin(theta_3) - ...
        cos(theta_2)*cos(theta_3)*sin(theta_1)) + ...
        sin(theta_4)*(cos(theta_2)*sin(theta_1)*sin(theta_3) + ...
        cos(theta_3)*sin(theta_1)*sin(theta_2))))/500, ...
        ...
        0; ...
    0, ...
        ...
        (39243*sin(theta_2)*sin(theta_3))/100000 - ...
        (39243*cos(theta_2)*cos(theta_3))/100000 - ...
        (17*cos(theta_2))/40 - ...
        (41*sin(theta_5)*(cos(theta_4)*(cos(theta_2)*cos(theta_3) - ...
        sin(theta_2)*sin(theta_3)) - sin(theta_4)*(cos(theta_2)*sin(theta_3) + ...
        cos(theta_3)*sin(theta_2))))/500 + ...
        (93*cos(theta_4)*(cos(theta_2)*sin(theta_3) + ...
        cos(theta_3)*sin(theta_2)))/1000 + ...
        (93*sin(theta_4)*(cos(theta_2)*cos(theta_3) - sin(theta_2)*sin(theta_3)))/1000,...
        ...
        (39243*sin(theta_2)*sin(theta_3))/100000 - ...
        (39243*cos(theta_2)*cos(theta_3))/100000 - ...
        (41*sin(theta_5)*(cos(theta_4)*(cos(theta_2)*cos(theta_3) - ...
        sin(theta_2)*sin(theta_3)) - sin(theta_4)*(cos(theta_2)*sin(theta_3) + ...
        cos(theta_3)*sin(theta_2))))/500 + (93*cos(theta_4)*(cos(theta_2)*sin(theta_3) + ...
        cos(theta_3)*sin(theta_2)))/1000 + (93*sin(theta_4)*(cos(theta_2)*cos(theta_3) - ...
        sin(theta_2)*sin(theta_3)))/1000, ...
        ...
        (93*cos(theta_4)*(cos(theta_2)*sin(theta_3) + cos(theta_3)*sin(theta_2)))/1000 - ...
        (41*sin(theta_5)*(cos(theta_4)*(cos(theta_2)*cos(theta_3) - ...
        sin(theta_2)*sin(theta_3)) - sin(theta_4)*(cos(theta_2)*sin(theta_3) + ...
        cos(theta_3)*sin(theta_2))))/500 + (93*sin(theta_4)*(cos(theta_2)*cos(theta_3) - ...
        sin(theta_2)*sin(theta_3)))/1000,  ...
        ...
        -(41*cos(theta_5)*(cos(theta_4)*(cos(theta_2)*sin(theta_3) + ...
        cos(theta_3)*sin(theta_2)) + sin(theta_4)*(cos(theta_2)*cos(theta_3) - ...
        sin(theta_2)*sin(theta_3))))/500,  ...
        ...
        0; ...
    0, ...
        ...
        sin(theta_1), ...
        ...
        sin(theta_1), ...
        ...
        sin(theta_1), ...
        ...
        cos(theta_4)*(cos(theta_1)*cos(theta_2)*sin(theta_3) + ...
        cos(theta_1)*cos(theta_3)*sin(theta_2)) - ...
        sin(theta_4)*(cos(theta_1)*sin(theta_2)*sin(theta_3) - ...
        cos(theta_1)*cos(theta_2)*cos(theta_3)), ...
        ...
        cos(theta_5)*sin(theta_1) + ...
        sin(theta_5)*(cos(theta_4)*(cos(theta_1)*sin(theta_2)*sin(theta_3) - ...
        cos(theta_1)*cos(theta_2)*cos(theta_3)) + ...
        sin(theta_4)*(cos(theta_1)*cos(theta_2)*sin(theta_3) + ...
        cos(theta_1)*cos(theta_3)*sin(theta_2)));...
    0, ...
        ...
        -cos(theta_1), ...
        ...
        -cos(theta_1), ...
        ...
        -cos(theta_1), ...
        ...
        cos(theta_4)*(cos(theta_2)*sin(theta_1)*sin(theta_3) + ...
        cos(theta_3)*sin(theta_1)*sin(theta_2)) - ...
        sin(theta_4)*(sin(theta_1)*sin(theta_2)*sin(theta_3) - ...
        cos(theta_2)*cos(theta_3)*sin(theta_1)), ...
        ...
        sin(theta_5)*(cos(theta_4)*(sin(theta_1)*sin(theta_2)*sin(theta_3) - ...
        cos(theta_2)*cos(theta_3)*sin(theta_1)) + ...
        sin(theta_4)*(cos(theta_2)*sin(theta_1)*sin(theta_3) + ...
        cos(theta_3)*sin(theta_1)*sin(theta_2))) - cos(theta_1)*cos(theta_5);
    1, ...
        ...
        0, ...
        ...
        0, ...
        ...
        0, ...
        ...
        sin(theta_4)*(cos(theta_2)*sin(theta_3) + cos(theta_3)*sin(theta_2)) - ...
        cos(theta_4)*(cos(theta_2)*cos(theta_3) - sin(theta_2)*sin(theta_3)),...
        ...
        -sin(theta_5)*(cos(theta_4)*(cos(theta_2)*sin(theta_3) + ...
        cos(theta_3)*sin(theta_2)) + sin(theta_4)*(cos(theta_2)*cos(theta_3) - ...
        sin(theta_2)*sin(theta_3)));];
    
    tcp_speed = J*dq;

end

== matlab function JointSpaceControl_BestInertia/Forward & Velocity Kinematics Joint -> Tool Geometric Jacobian/J (made by Kathi) ==
  data: J output; q input; J1 output; J2 output
function [J, J1, J2]    = Jacobian(q)
% JACOBIAN - Jacobian from Base to Tool.
%  Calculates the Base-Tool Transformation matrix based on the current
%  joint positions and returns the rotation matrix and the displacement
%  vector.

theta_1 = q(1);
theta_2 = q(2);
theta_3 = q(3);
theta_4 = q(4);
theta_5 = q(5);
theta_6 = q(6);

J = [(109*cos(theta_1))/1000 + (41*cos(theta_1)*cos(theta_5))/500 + ...
        (17*cos(theta_2)*sin(theta_1))/40 - ...
        (93*cos(theta_4)*(cos(theta_2)*sin(theta_1)*sin(theta_3) + ...
        cos(theta_3)*sin(theta_1)*sin(theta_2)))/1000 + ...
        (93*sin(theta_4)*(sin(theta_1)*sin(theta_2)*sin(theta_3) - ...
        cos(theta_2)*cos(theta_3)*sin(theta_1)))/1000 - ...
        (41*sin(theta_5)*(cos(theta_4)*(sin(theta_1)*sin(theta_2)*sin(theta_3) - ...
        cos(theta_2)*cos(theta_3)*sin(theta_1)) + ...
        sin(theta_4)*(cos(theta_2)*sin(theta_1)*sin(theta_3) + ...
        cos(theta_3)*sin(theta_1)*sin(theta_2))))/500 - ...
        (39243*sin(theta_1)*sin(theta_2)*sin(theta_3))/100000 + ...
        (39243*cos(theta_2)*cos(theta_3)*sin(theta_1))/100000, ...
        ...
        (17*cos(theta_1)*sin(theta_2))/40 - ...
        (93*cos(theta_4)*(cos(theta_1)*sin(theta_2)*sin(theta_3) - ...
        cos(theta_1)*cos(theta_2)*cos(theta_3)))/1000 - ...
        (93*sin(theta_4)*(cos(theta_1)*cos(theta_2)*sin(theta_3) + ...
        cos(theta_1)*cos(theta_3)*sin(theta_2)))/1000 + ...
        (41*sin(theta_5)*(cos(theta_4)*(cos(theta_1)*cos(theta_2)*sin(theta_3) + ...
        cos(theta_1)*cos(theta_3)*sin(theta_2)) - ...
        sin(theta_4)*(cos(theta_1)*sin(theta_2)*sin(theta_3) - ...
        cos(theta_1)*cos(theta_2)*cos(theta_3))))/500 + ...
        (39243*cos(theta_1)*cos(theta_2)*sin(theta_3))/100000 + ...
        (39243*cos(theta_1)*cos(theta_3)*sin(theta_2))/100000, ...
        ...
        (41*sin(theta_5)*(cos(theta_4)*(cos(theta_1)*cos(theta_2)*sin(theta_3) + ...
        cos(theta_1)*cos(theta_3)*sin(theta_2)) - ...
        sin(theta_4)*(cos(theta_1)*sin(theta_2)*sin(theta_3) - ...
        cos(theta_1)*cos(theta_2)*cos(theta_3))))/500 - ...
        (93*sin(theta_4)*(cos(theta_1)*cos(theta_2)*sin(theta_3) + ...
        cos(theta_1)*cos(theta_3)*sin(theta_2)))/1000 - ...
        (93*cos(theta_4)*(cos(theta_1)*sin(theta_2)*sin(theta_3) - ...
        cos(theta_1)*cos(theta_2)*cos(theta_3)))/1000 + ...
        (39243*cos(theta_1)*cos(theta_2)*sin(theta_3))/100000 + ...
        (39243*cos(theta_1)*cos(theta_3)*sin(theta_2))/100000, ...
        ...
        (41*sin(theta_5)*(cos(theta_4)*(cos(theta_1)*cos(theta_2)*sin(theta_3) + ...
        cos(theta_1)*cos(theta_3)*sin(theta_2)) - ...
        sin(theta_4)*(cos(theta_1)*sin(theta_2)*sin(theta_3) - ...
        cos(theta_1)*cos(theta_2)*cos(theta_3))))/500 - ...
        (93*sin(theta_4)*(cos(theta_1)*cos(theta_2)*sin(theta_3) + ...
        cos(theta_1)*cos(theta_3)*sin(theta_2)))/1000 - ...
        (93*cos(theta_4)*(cos(theta_1)*sin(theta_2)*sin(theta_3) - ...
        cos(theta_1)*cos(theta_2)*cos(theta_3)))/1000, ...
        ...
        (41*cos(theta_5)*(cos(theta_4)*(cos(theta_1)*sin(theta_2)*sin(theta_3) - ...
        cos(theta_1)*cos(theta_2)*cos(theta_3)) + ...
        sin(theta_4)*(cos(theta_1)*cos(theta_2)*sin(theta_3) + ...
        cos(theta_1)*cos(theta_3)*sin(theta_2))))/500 - ...
        (41*sin(theta_1)*sin(theta_5))/500,... 
        ...
        0; ...
   (109*sin(theta_1))/1000 - (17*cos(theta_1)*cos(theta_2))/40 + ...
        (41*cos(theta_5)*sin(theta_1))/500 + ...
        (93*cos(theta_4)*(cos(theta_1)*cos(theta_2)*sin(theta_3) + ...
        cos(theta_1)*cos(theta_3)*sin(theta_2)))/1000 - ...
        (93*sin(theta_4)*(cos(theta_1)*sin(theta_2)*sin(theta_3) - ... 
        cos(theta_1)*cos(theta_2)*cos(theta_3)))/1000 + ...
        (41*sin(theta_5)*(cos(theta_4)*(cos(theta_1)*sin(theta_2)*sin(theta_3) - ...
        cos(theta_1)*cos(theta_2)*cos(theta_3)) + ...
        sin(theta_4)*(cos(theta_1)*cos(theta_2)*sin(theta_3) + ...
        cos(theta_1)*cos(theta_3)*sin(theta_2))))/500 + ...
        (39243*cos(theta_1)*sin(theta_2)*sin(theta_3))/100000 - ...
        (39243*cos(theta_1)*cos(theta_2)*cos(theta_3))/100000, ...
        ...
        (17*sin(theta_1)*sin(theta_2))/40 - ...
        (93*cos(theta_4)*(sin(theta_1)*sin(theta_2)*sin(theta_3) - ...
        cos(theta_2)*cos(theta_3)*sin(theta_1)))/1000 - ...
        (93*sin(theta_4)*(cos(theta_2)*sin(theta_1)*sin(theta_3) + ...
        cos(theta_3)*sin(theta_1)*sin(theta_2)))/1000 + ...
        (41*sin(theta_5)*(cos(theta_4)*(cos(theta_2)*sin(theta_1)*sin(theta_3) + ...
        cos(theta_3)*sin(theta_1)*sin(theta_2)) - ...
        sin(theta_4)*(sin(theta_1)*sin(theta_2)*sin(theta_3) - ...
        cos(theta_2)*cos(theta_3)*sin(theta_1))))/500 + ...
        (39243*cos(theta_2)*sin(theta_1)*sin(theta_3))/100000 + ...
        (39243*cos(theta_3)*sin(theta_1)*sin(theta_2))/100000, ...
        ...
        (41*sin(theta_5)*(cos(theta_4)*(cos(theta_2)*sin(theta_1)*sin(theta_3) + ...
        cos(theta_3)*sin(theta_1)*sin(theta_2)) - ...
        sin(theta_4)*(sin(theta_1)*sin(theta_2)*sin(theta_3) - ...
        cos(theta_2)*cos(theta_3)*sin(theta_1))))/500 - ...
        (93*sin(theta_4)*(cos(theta_2)*sin(theta_1)*sin(theta_3) + ...
        cos(theta_3)*sin(theta_1)*sin(theta_2)))/1000 - ...
        (93*cos(theta_4)*(sin(theta_1)*sin(theta_2)*sin(theta_3) - ...
        cos(theta_2)*cos(theta_3)*sin(theta_1)))/1000 + ...
        (39243*cos(theta_2)*sin(theta_1)*sin(theta_3))/100000 + ...
        (39243*cos(theta_3)*sin(theta_1)*sin(theta_2))/100000, ...
        ...
        (41*sin(theta_5)*(cos(theta_4)*(cos(theta_2)*sin(theta_1)*sin(theta_3) + ...
        cos(theta_3)*sin(theta_1)*sin(theta_2)) - ...
        sin(theta_4)*(sin(theta_1)*sin(theta_2)*sin(theta_3) - ...
        cos(theta_2)*cos(theta_3)*sin(theta_1))))/500 - ...
        (93*sin(theta_4)*(cos(theta_2)*sin(theta_1)*sin(theta_3) + ...
        cos(theta_3)*sin(theta_1)*sin(theta_2)))/1000 - ...
        (93*cos(theta_4)*(sin(theta_1)*sin(theta_2)*sin(theta_3) - ...
        cos(theta_2)*cos(theta_3)*sin(theta_1)))/1000, ...
        ...
        (41*cos(theta_1)*sin(theta_5))/500 + ...
        (41*cos(theta_5)*(cos(theta_4)*(sin(theta_1)*sin(theta_2)*sin(theta_3) - ...
        cos(theta_2)*cos(theta_3)*sin(theta_1)) + ...
        sin(theta_4)*(cos(theta_2)*sin(theta_1)*sin(theta_3) + ...
        cos(theta_3)*sin(theta_1)*sin(theta_2))))/500, ...
        ...
        0; ...
    0, ...
        ...
        (39243*sin(theta_2)*sin(theta_3))/100000 - ...
        (39243*cos(theta_2)*cos(theta_3))/100000 - ...
        (17*cos(theta_2))/40 - ...
        (41*sin(theta_5)*(cos(theta_4)*(cos(theta_2)*cos(theta_3) - ...
        sin(theta_2)*sin(theta_3)) - sin(theta_4)*(cos(theta_2)*sin(theta_3) + ...
        cos(theta_3)*sin(theta_2))))/500 + ...
        (93*cos(theta_4)*(cos(theta_2)*sin(theta_3) + ...
        cos(theta_3)*sin(theta_2)))/1000 + ...
        (93*sin(theta_4)*(cos(theta_2)*cos(theta_3) - sin(theta_2)*sin(theta_3)))/1000,...
        ...
        (39243*sin(theta_2)*sin(theta_3))/100000 - ...
        (39243*cos(theta_2)*cos(theta_3))/100000 - ...
        (41*sin(theta_5)*(cos(theta_4)*(cos(theta_2)*cos(theta_3) - ...
        sin(theta_2)*sin(theta_3)) - sin(theta_4)*(cos(theta_2)*sin(theta_3) + ...
        cos(theta_3)*sin(theta_2))))/500 + (93*cos(theta_4)*(cos(theta_2)*sin(theta_3) + ...
        cos(theta_3)*sin(theta_2)))/1000 + (93*sin(theta_4)*(cos(theta_2)*cos(theta_3) - ...
        sin(theta_2)*sin(theta_3)))/1000, ...
        ...
        (93*cos(theta_4)*(cos(theta_2)*sin(theta_3) + cos(theta_3)*sin(theta_2)))/1000 - ...
        (41*sin(theta_5)*(cos(theta_4)*(cos(theta_2)*cos(theta_3) - ...
        sin(theta_2)*sin(theta_3)) - sin(theta_4)*(cos(theta_2)*sin(theta_3) + ...
        cos(theta_3)*sin(theta_2))))/500 + (93*sin(theta_4)*(cos(theta_2)*cos(theta_3) - ...
        sin(theta_2)*sin(theta_3)))/1000,  ...
        ...
        -(41*cos(theta_5)*(cos(theta_4)*(cos(theta_2)*sin(theta_3) + ...
        cos(theta_3)*sin(theta_2)) + sin(theta_4)*(cos(theta_2)*cos(theta_3) - ...
        sin(theta_2)*sin(theta_3))))/500,  ...
        ...
        0; ...
    0, ...
        ...
        sin(theta_1), ...
        ...
        sin(theta_1), ...
        ...
        sin(theta_1), ...
        ...
        cos(theta_4)*(cos(theta_1)*cos(theta_2)*sin(theta_3) + ...
        cos(theta_1)*cos(theta_3)*sin(theta_2)) - ...
        sin(theta_4)*(cos(theta_1)*sin(theta_2)*sin(theta_3) - ...
        cos(theta_1)*cos(theta_2)*cos(theta_3)), ...
        ...
        cos(theta_5)*sin(theta_1) + ...
        sin(theta_5)*(cos(theta_4)*(cos(theta_1)*sin(theta_2)*sin(theta_3) - ...
        cos(theta_1)*cos(theta_2)*cos(theta_3)) + ...
        sin(theta_4)*(cos(theta_1)*cos(theta_2)*sin(theta_3) + ...
        cos(theta_1)*cos(theta_3)*sin(theta_2)));...
    0, ...
        ...
        -cos(theta_1), ...
        ...
        -cos(theta_1), ...
        ...
        -cos(theta_1), ...
        ...
        cos(theta_4)*(cos(theta_2)*sin(theta_1)*sin(theta_3) + ...
        cos(theta_3)*sin(theta_1)*sin(theta_2)) - ...
        sin(theta_4)*(sin(theta_1)*sin(theta_2)*sin(theta_3) - ...
        cos(theta_2)*cos(theta_3)*sin(theta_1)), ...
        ...
        sin(theta_5)*(cos(theta_4)*(sin(theta_1)*sin(theta_2)*sin(theta_3) - ...
        cos(theta_2)*cos(theta_3)*sin(theta_1)) + ...
        sin(theta_4)*(cos(theta_2)*sin(theta_1)*sin(theta_3) + ...
        cos(theta_3)*sin(theta_1)*sin(theta_2))) - cos(theta_1)*cos(theta_5);
    1, ...
        ...
        0, ...
        ...
        0, ...
        ...
        0, ...
        ...
        sin(theta_4)*(cos(theta_2)*sin(theta_3) + cos(theta_3)*sin(theta_2)) - ...
        cos(theta_4)*(cos(theta_2)*cos(theta_3) - sin(theta_2)*sin(theta_3)),...
        ...
        -sin(theta_5)*(cos(theta_4)*(cos(theta_2)*sin(theta_3) + ...
        cos(theta_3)*sin(theta_2)) + sin(theta_4)*(cos(theta_2)*cos(theta_3) - ...
        sin(theta_2)*sin(theta_3)));];
    J1 = J(1:6,1:3);
    J2 = J(1:6,4:6); 

end
